simulink model "PMSM_Linear_vs_NaoLinear"  (R2021a)
settings: Solver=ode1  StartTime=0.0  StopTime=0.6  FixedStep=1e-6  RelTol=1e-3
undefined symbols (not defined in the file or in its folder): A, B, id, iq, Vd, Vq, w
settings Model: Creator=migue  LastModifiedBy=migue

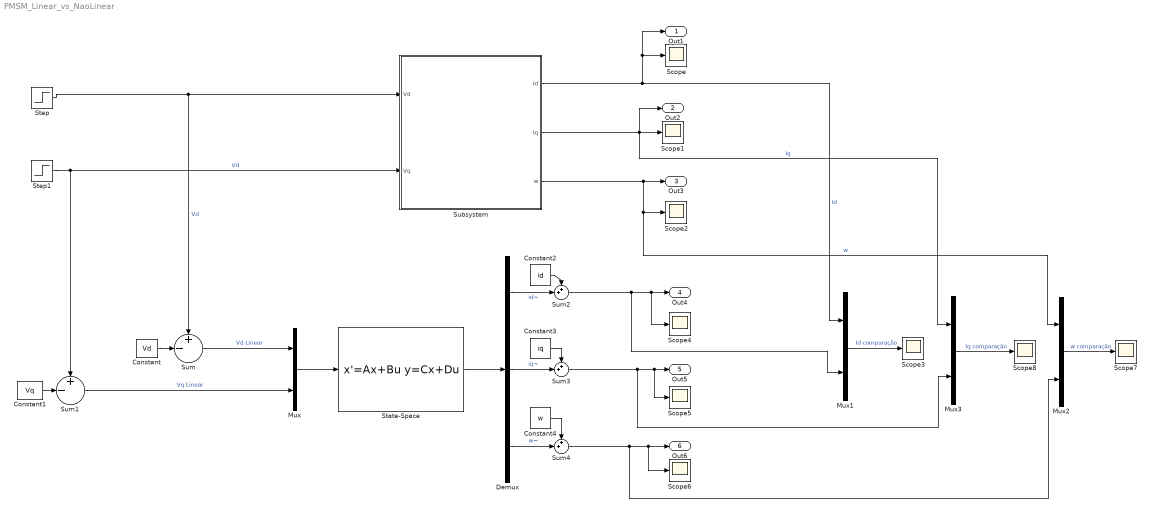
== system PMSM_Linear_vs_NaoLinear ==
  Constant : Constant  Value=Vd
  Constant1 : Constant  Value=Vq
  Constant2 : Constant  Value=id
  Constant3 : Constant  Value=iq
  Constant4 : Constant  Value=w
  Demux : Demux  Outputs=3
  Mux{,1..3} (4 alike) : Mux  Inputs=2
  Scope{,1..8} (9 alike) : Scope
  State-Space : StateSpace  A=A  B=B  C=eye(3)  D=zeros(3,2)  InitialCondition=zeros(3,1)
  Step : Step  Time=0.5  Before=Vd  After=Vd*1.1  SampleTime=0
  Step1 : Step  Time=0.5  Before=Vq  After=Vq*1.1  SampleTime=0
  Subsystem : Subsystem  mask{R=0.16, L=1.3e-4, N=10, J=1.8e-4, b=1e-5, lamb=0.06, Kt=0.095}
      mask prompts: R "Resitência (R)"; L "Indutância(L)"; N "Nº de par de polos(N)"; J "coeficiente(J)"; b "coeficiente(b)"; lamb "(lamb)"; Kt "(Kt)"
  Sum : Sum  Inputs=+-|
  Sum1 : Sum  Inputs=+-|
  Sum2 : Sum  Inputs=++|
  Sum3 : Sum  Inputs=++|
  Sum4 : Sum  Inputs=++|
  Out1 : Outport
  Out2 : Outport  Port=2
  Out3 : Outport  Port=3
  Out4 : Outport  Port=4
  Out5 : Outport  Port=5
  Out6 : Outport  Port=6
  wires:
  Subsystem/1(Id) -> Mux1/1, Out1/1, Scope/1  "Id"
  Subsystem/2(Iq) -> Out2/1, Scope1/1, Mux3/1  "Iq"
  Subsystem/3(w) -> Mux2/1, Scope2/1, Out3/1  "w"
  Step/1 -> Sum/1, Subsystem/1(Vd)  "Vd"
  Step1/1 -> Subsystem/2(Vq), Sum1/1  "Vd"
  Mux/1 -> State-Space/1
  State-Space/1 -> Demux/1
  Sum/1 -> Mux/1  "Vd Linear"
  Sum1/1 -> Mux/2  "Vq Linear"
  Constant1/1 -> Sum1/2
  Sum2/1 -> Mux1/2, Scope4/1, Out4/1
  Demux/1 -> Sum2/2  "id~"
  Constant2/1 -> Sum2/1
  Constant3/1 -> Sum3/1
  Demux/2 -> Sum3/2  "iq~"
  Sum3/1 -> Mux3/2, Scope5/1, Out5/1
  Constant4/1 -> Sum4/1
  Demux/3 -> Sum4/2  "w~"
  Sum4/1 -> Mux2/2, Out6/1, Scope6/1
  Mux2/1 -> Scope7/1  "w comparação"
  Mux3/1 -> Scope8/1  "Iq comparação"
  Mux1/1 -> Scope3/1  "Id comparação"
  Constant/1 -> Sum/2

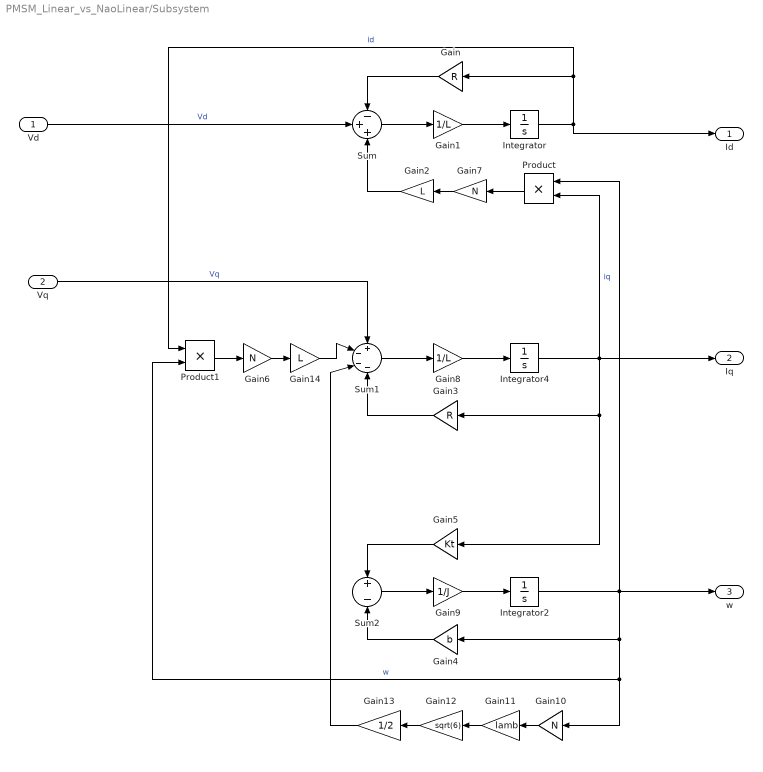
== system PMSM_Linear_vs_NaoLinear/Subsystem ==
  Vd : Inport
  Vq : Inport  Port=2
  Gain : Gain  Gain=R
  Gain1 : Gain  Gain=1/L
  Gain10 : Gain  Gain=N
  Gain11 : Gain  Gain=lamb
  Gain12 : Gain  Gain=sqrt(6)
  Gain13 : Gain  Gain=1/2
  Gain14 : Gain  Gain=L
  Gain2 : Gain  Gain=L
  Gain3 : Gain  Gain=R
  Gain4 : Gain  Gain=b
  Gain5 : Gain  Gain=Kt
  Gain6 : Gain  Gain=N
  Gain7 : Gain  Gain=N
  Gain8 : Gain  Gain=1/L
  Gain9 : Gain  Gain=1/J
  Integrator : Integrator  InitialCondition=id
  Integrator2 : Integrator  InitialCondition=w
  Integrator4 : Integrator  InitialCondition=iq
  Product : Product
  Product1 : Product
  Sum : Sum  Inputs=-++
  Sum1 : Sum  Inputs=+---
  Sum2 : Sum  Inputs=+-
  Id : Outport
  Iq : Outport  Port=2
  w : Outport  Port=3
  wires:
  Integrator4/1 -> Iq/1, Product/2, Gain3/1, Gain5/1  "iq"
  Integrator/1 -> Gain/1, Product1/1, Id/1  "id"
  Gain8/1 -> Integrator4/1
  Sum1/1 -> Gain8/1
  Product1/1 -> Gain6/1
  Gain/1 -> Sum/1
  Sum2/1 -> Gain9/1
  Integrator2/1 -> w/1, Product/1, Gain10/1, Product1/2, Gain4/1  "w"
  Gain5/1 -> Sum2/1
  Vd/1 -> Sum/2  "Vd"
  Gain9/1 -> Integrator2/1
  Gain1/1 -> Integrator/1
  Sum/1 -> Gain1/1
  Gain4/1 -> Sum2/2
  Gain3/1 -> Sum1/4
  Gain11/1 -> Gain12/1
  Gain10/1 -> Gain11/1
  Product/1 -> Gain7/1
  Vq/1 -> Sum1/1  "Vq"
  Gain12/1 -> Gain13/1
  Gain13/1 -> Sum1/3
  Gain6/1 -> Gain14/1
  Gain7/1 -> Gain2/1
  Gain2/1 -> Sum/3
  Gain14/1 -> Sum1/2
